simulink model "sim_flexible_unsteady_indi_turbulence"  (R2018b)
settings: Solver=ode4  StartTime=0.0  StopTime=12  FixedStep=1/600  RelTol=1e-2  AbsTol=1e-2
model workspace (MAT data in the model file):
  Var = 0
undefined symbols (not defined in the file): aircraft, alt_ground, atmosphere, envir, g, gla_indi, ic, jystck
libraries: simulink x3, atmosphere_lib x2, se2a_controller_lib x2, InputBlocks_library x2, flight_dynamics_models x1, sensors_lib x1, se2a_command_lib x1, joystick_lib x1, dspnetwork x1, flexiFlightVis_lib x1, aeroelasticity_lib x1
settings Model: EnablePacing=on  PacingRate=0.100000  ParamWorkspaceSource=ReferencedWorkspace  TunableVars=test_val  TunableVarsStorageClass=ExportedGlobal  Creator=Yannic  LastModifiedBy=yannic
settings DataIOCC: ExternalInput=[0,tp_indi.Input']  InitialState=tp_indi.State  LoadExternalInput=on  LoadInitialState=on

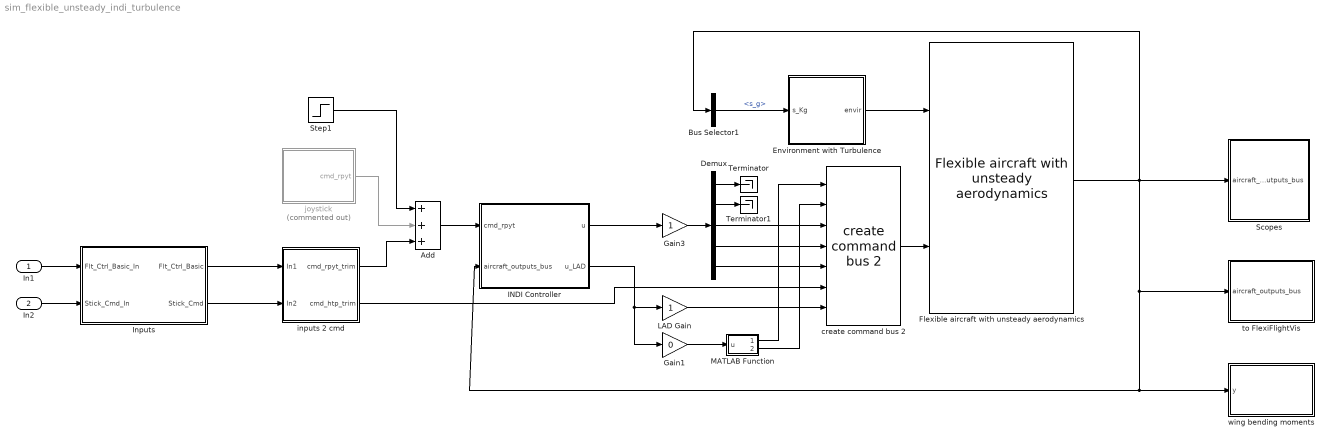
== system sim_flexible_unsteady_indi_turbulence ==
  In1 : Inport
  In2 : Inport  Port=2
  Add : Sum  Inputs=+++
  Bus Selector1 : BusSelector  OutputSignals=flexible_body_bus.rigidBodyBus.s_g
  Demux : Demux  Outputs=5
  Environment with Turbulence : Subsystem  mask{envir=envir, wind_input=2, F_g=0, gustGradDist=100, Delta_gustGradDist=100, Delta_time=3, time_0=1}
      mask prompts: envir "environment struct"; wind_input "Switch wing model (1=disable, 2=1-cos gust)"; F_g "Flight profile alleviation factor"; gustGradDist "Initial gust gradient distance, in ft"; Delta_gustGradDist "Delta gust gradient distance, in ft"; Delta_time "Time between gusts, in s"; time_0 "Time of first gust, in s"
      mask DialogControl DescGroupVar Prompt: Environment with successive 1-cos gusts
      mask DialogControl DescTextVar Prompt: Note that for the local gust delays the following structs must be in the base workspace: wing_main, wing_htp, wing_vtp, fuselage
  Flexible aircraft with unsteady aerodynamics : flight_dynamics_models/Flexible aircraft with unsteady aerodynamics  aircraft=aircraft  ic=ic
      settings: SourceProductName=SE2A library
  Gain1 : Gain  Gain=0
  Gain3 : Gain
  INDI Controller : Subsystem
  Inputs : Subsystem
  LAD Gain : Gain
  MATLAB Function : MATLAB Function  TreatAsAtomicUnit=on
  Scopes : Subsystem
  Step1 : Step  Before=zeros(4,1)  After=[0;0.05;0;0]*0  SampleTime=0
  Terminator : Terminator
  Terminator1 : Terminator
  create command bus 2 : se2a_command_lib/create command bus 2
      settings: SourceProductName=SE2A library
  inputs 2 cmd : Subsystem
  joystick : Subsystem  Commented=on
  to FlexiFlightVis : Subsystem
  wing bending moments : Subsystem
  wires:
  Environment with Turbulence/1(envir) -> Flexible aircraft with unsteady aerodynamics/1
  create command bus 2/1 -> Flexible aircraft with unsteady aerodynamics/2
  Bus Selector1/1 -> Environment with Turbulence/1(s_Kg)  "<s_g>"
  Flexible aircraft with unsteady aerodynamics/1 -> to FlexiFlightVis/1(aircraft_outputs_bus), INDI Controller/2(aircraft_outputs_bus), wing bending moments/1(y), Scopes/1(aircraft_outputs_bus), Bus Selector1/1
  joystick/1(cmd_rpyt) -> Add/2
  Demux/1 -> Terminator/1
  Demux/2 -> Terminator1/1
  Demux/3 -> create command bus 2/3
  Demux/4 -> create command bus 2/4
  Demux/5 -> create command bus 2/5
  inputs 2 cmd/2(cmd_htp_trim) -> create command bus 2/6
  In1/1 -> Inputs/1(Flt_Ctrl_Basic_In)
  In2/1 -> Inputs/2(Stick_Cmd_In)
  Inputs/1(Flt_Ctrl_Basic) -> inputs 2 cmd/1(In1)
  Inputs/2(Stick_Cmd) -> inputs 2 cmd/2(In2)
  Add/1 -> INDI Controller/1(cmd_rpyt)
  inputs 2 cmd/1(cmd_rpyt_trim) -> Add/3
  INDI Controller/1(u) -> Gain3/1
  Gain3/1 -> Demux/1
  INDI Controller/2(u_LAD) -> Gain1/1, LAD Gain/1
  MATLAB Function/1(a_l) -> create command bus 2/1
  MATLAB Function/2(a_r) -> create command bus 2/2
  Step1/1 -> Add/1
  Gain1/1 -> MATLAB Function/1(u)
  LAD Gain/1 -> create command bus 2/7

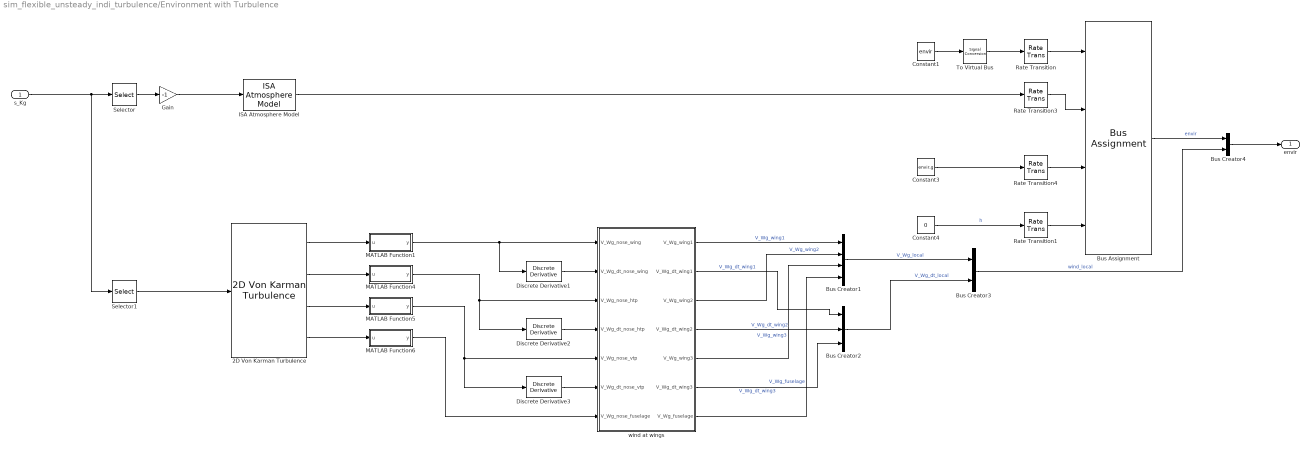
== system sim_flexible_unsteady_indi_turbulence/Environment with Turbulence ==
  s_Kg : Inport
  2D Von Karman Turbulence : atmosphere_lib/2D Von Karman Turbulence  x_max=10000  y_max=2*762  Delta_x=1  Delta_y=1  sigma=6.5  L=762  Y={aircraft.wing_main.geometry.ctrl_pt.pos(2,:),aircraft.wing_htp.geometry.ctrl_pt.pos(2,:),aircraft.wing_vtp.geometry.ctrl_pt.pos(2,:),0}  is_symmetric=on  seed=2
      settings: SourceProductName=LADAC
  Bus Assignment : BusAssignment  AssignedSignals=atmosphere,g,alt_ground
  Bus Creator1 : BusCreator  Inputs=4
  Bus Creator2 : BusCreator  Inputs=3
  Bus Creator3 : BusCreator  Inputs=2
  Bus Creator4 : BusCreator  Inputs=2
  Constant1 : Constant  Value=envir  OutDataTypeStr=Bus: envirBus
  Constant3 : Constant  Value=envir.g
  Constant4 : Constant  Value=0
  Discrete Derivative1 : simulink/Discrete/Discrete Derivative  gainval=1.0  ICPrevScaledInput=0.0  OutMin=[]  OutMax=[]  OutDataType=fixdt(1, 16)  OutScaling=2^-10  DoSatur=off
  Discrete Derivative2 : simulink/Discrete/Discrete Derivative  gainval=1.0  ICPrevScaledInput=0.0  OutMin=[]  OutMax=[]  OutDataType=fixdt(1, 16)  OutScaling=2^-10  DoSatur=off
  Discrete Derivative3 : simulink/Discrete/Discrete Derivative  gainval=1.0  ICPrevScaledInput=0.0  OutMin=[]  OutMax=[]  OutDataType=fixdt(1, 16)  OutScaling=2^-10  DoSatur=off
  Gain : Gain  Gain=-1
  ISA Atmosphere Model : atmosphere_lib/ISA Atmosphere Model
      settings: SourceProductName=LADAC
  MATLAB Function1 : MATLAB Function  TreatAsAtomicUnit=on
  MATLAB Function4 : MATLAB Function  TreatAsAtomicUnit=on
  MATLAB Function5 : MATLAB Function  TreatAsAtomicUnit=on
  MATLAB Function6 : MATLAB Function  TreatAsAtomicUnit=on
  Rate Transition{,1,3..4} (4 alike) : RateTransition
  Selector : Selector  InputPortWidth=3  IndexOptions=Index vector (dialog)  Indices=3  OutputSizes=1
  Selector1 : Selector  InputPortWidth=3  IndexOptions=Index vector (dialog)  Indices=1  OutputSizes=1
  To Virtual Bus : SignalConversion  ConversionOutput=Virtual bus  OverrideOpt=off
  wind at wings : Subsystem  mask{aircraft=aircraft, V_A=norm(ic.V_Kb,2)}
      mask prompts: aircraft "Aircraft parameters struct, see aircraftSe2aCreate"; V_A "Airspeed (TAS) in m/s"
      mask init:
      | Delta_time_main_wing = abs(aircraft.wing_main.params.x+aircraft.wing_main.geometry.ctrl_pt.pos(1,:))/V_A;
      | Delta_time_htp = abs(aircraft.wing_htp.params.x+aircraft.wing_htp.geometry.ctrl_pt.pos(1,:))/V_A;
      | Delta_time_vtp = abs(aircraft.wing_vtp.params.x+aircraft.wing_vtp.geometry.ctrl_pt.pos(1,:))/V_A;
      | Delta_time_fuse = abs(aircraft.fuselage.geometry.border_pos(1,:))/V_A;
  envir : Outport
  wires:
  wind at wings/7(V_Wg_fuselage) -> Bus Creator1/4  "V_Wg_fuselage"
  Selector/1 -> Gain/1
  s_Kg/1 -> Selector1/1, Selector/1
  To Virtual Bus/1 -> Rate Transition/1
  Bus Creator4/1 -> envir/1
  Bus Creator3/1 -> Bus Creator4/2  "wind_local"
  Bus Creator2/1 -> Bus Creator3/2  "V_Wg_dt_local"
  wind at wings/2(V_Wg_dt_wing1) -> Bus Creator2/1  "V_Wg_dt_wing1"
  wind at wings/4(V_Wg_dt_wing2) -> Bus Creator2/2  "V_Wg_dt_wing2"
  wind at wings/6(V_Wg_dt_wing3) -> Bus Creator2/3  "V_Wg_dt_wing3"
  Bus Creator1/1 -> Bus Creator3/1  "V_Wg_local"
  wind at wings/5(V_Wg_wing3) -> Bus Creator1/3  "V_Wg_wing3"
  wind at wings/3(V_Wg_wing2) -> Bus Creator1/2  "V_Wg_wing2"
  wind at wings/1(V_Wg_wing1) -> Bus Creator1/1  "V_Wg_wing1"
  Constant3/1 -> Rate Transition4/1
  Rate Transition4/1 -> Bus Assignment/3
  Gain/1 -> ISA Atmosphere Model/1
  Constant1/1 -> To Virtual Bus/1
  Rate Transition1/1 -> Bus Assignment/4
  ISA Atmosphere Model/1 -> Rate Transition3/1
  Rate Transition/1 -> Bus Assignment/1
  Bus Assignment/1 -> Bus Creator4/1  "envir"
  Rate Transition3/1 -> Bus Assignment/2
  Constant4/1 -> Rate Transition1/1  "h"
  Selector1/1 -> 2D Von Karman Turbulence/1
  2D Von Karman Turbulence/1 -> MATLAB Function1/1(u)
  MATLAB Function1/1(y) -> wind at wings/1(V_Wg_nose_wing), Discrete Derivative1/1
  Discrete Derivative1/1 -> wind at wings/2(V_Wg_dt_nose_wing)
  2D Von Karman Turbulence/2 -> MATLAB Function4/1(u)
  MATLAB Function4/1(y) -> Discrete Derivative2/1, wind at wings/3(V_Wg_nose_htp)
  2D Von Karman Turbulence/3 -> MATLAB Function5/1(u)
  MATLAB Function5/1(y) -> wind at wings/5(V_Wg_nose_vtp), Discrete Derivative3/1
  2D Von Karman Turbulence/4 -> MATLAB Function6/1(u)
  MATLAB Function6/1(y) -> wind at wings/7(V_Wg_nose_fuselage)
  Discrete Derivative2/1 -> wind at wings/4(V_Wg_dt_nose_htp)
  Discrete Derivative3/1 -> wind at wings/6(V_Wg_dt_nose_vtp)

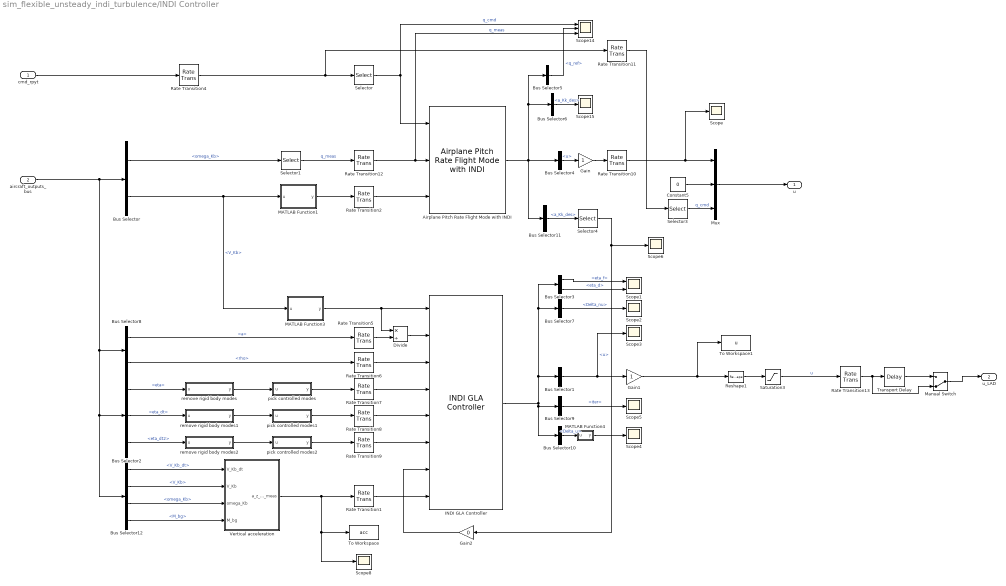
== system sim_flexible_unsteady_indi_turbulence/INDI Controller ==
  cmd_rpyt : Inport
  aircraft_outputs_bus : Inport  Port=2
  Airplane Pitch Rate Flight Mode with INDI : se2a_controller_lib/Airplane Pitch Rate Flight Mode with INDI  fm=pitch_rate_controller
  Bus Selector : BusSelector  OutputSignals=flexible_body_bus.rigidBodyBus.omega_Kb,flexible_body_bus.rigidBodyBus.V_Kb
  Bus Selector1 : BusSelector  OutputSignals=u
  Bus Selector10 : BusSelector  OutputSignals=Delta_u
  Bus Selector11 : BusSelector  OutputSignals=direct_lift_control.a_Kk_des
  Bus Selector12 : BusSelector  OutputSignals=flexible_body_bus.rigidBodyBus.V_Kb_dt,flexible_body_bus.rigidBodyBus.V_Kb,flexible_body_bus.rigidBodyBus.omega_Kb,flexible_body_bus.rigidBodyBus.M_bg
  Bus Selector2 : BusSelector  OutputSignals=flexible_body_bus.eta,flexible_body_bus.eta_dt,flexible_body_bus.eta_dt2
  Bus Selector3 : BusSelector  OutputSignals=measure.eta_f,desired.eta_d
  Bus Selector4 : BusSelector  OutputSignals=u
  Bus Selector5 : BusSelector  OutputSignals=pitch_rate_control.reference.q_ref
  Bus Selector6 : BusSelector  OutputSignals=direct_lift_control.a_Kk_des
  Bus Selector7 : BusSelector  OutputSignals=pseudo_cntrl.Delta_nu
  Bus Selector8 : BusSelector  OutputSignals=aeroBus.main.external.atmosphere.a,aeroBus.main.external.atmosphere.rho
  Bus Selector9 : BusSelector  OutputSignals=iter
  Constant5 : Constant  Value=0
  Divide : Product  Inputs=*/
  Gain : Gain
  Gain1 : Gain
  Gain2 : Gain  Gain=0
  INDI GLA Controller : se2a_controller_lib/INDI GLA Controller  gla_indi=gla_indi
  MATLAB Function1 : MATLAB Function  TreatAsAtomicUnit=on
  MATLAB Function3 : MATLAB Function  TreatAsAtomicUnit=on
  MATLAB Function4 : MATLAB Function  TreatAsAtomicUnit=on
  Manual Switch : ManualSwitch  CurrentSetting=0
  Mux : Mux  Inputs=3
  Rate Transition{1,5..9} (6 alike) : RateTransition  OutPortSampleTime=gla_indi.ts
  Rate Transition{2,4,10..13} (6 alike) : RateTransition
  Reshape1 : Reshape
  Saturation3 : Saturate  UpperLimit=gla_indi.ca.u_max  LowerLimit=gla_indi.ca.u_min
  Scope{,2..6,8,15} (8 alike) : Scope
  Scope1 : Scope  NumInputPorts=2
  Scope14 : Scope  NumInputPorts=3
  Selector : Selector  InputPortWidth=4  IndexOptions=Index vector (dialog)  Indices=2  OutputSizes=1
  Selector1 : Selector  InputPortWidth=3  IndexOptions=Index vector (dialog)  Indices=2  OutputSizes=1
  Selector3 : Selector  InputPortWidth=4  IndexOptions=Index vector (dialog)  Indices=4  OutputSizes=1
  Selector4 : Selector  InputPortWidth=3  IndexOptions=Index vector (dialog)  Indices=3  OutputSizes=1
  To Workspace : ToWorkspace  VariableName=acc  SaveFormat=Timeseries  SampleTime=-1
  To Workspace1 : ToWorkspace  VariableName=u  SaveFormat=Timeseries  SampleTime=-1
  Transport Delay : TransportDelay  DelayTime=gla_indi.ts  TransDelayFeedthrough=on
  Vertical acceleration : Subsystem
  pick controlled modes : MATLAB Function  TreatAsAtomicUnit=on
  pick controlled modes1 : MATLAB Function  TreatAsAtomicUnit=on
  pick controlled modes2 : MATLAB Function  TreatAsAtomicUnit=on
  remove rigid body modes : MATLAB Function  TreatAsAtomicUnit=on
  remove rigid body modes1 : MATLAB Function  TreatAsAtomicUnit=on
  remove rigid body modes2 : MATLAB Function  TreatAsAtomicUnit=on
  u : Outport
  u_LAD : Outport  Port=2
  wires:
  cmd_rpyt/1 -> Rate Transition4/1
  aircraft_outputs_bus/1 -> Bus Selector12/1, Bus Selector2/1, Bus Selector8/1, Bus Selector/1
  Bus Selector/1 -> Selector1/1  "<omega_Kb>"
  Bus Selector/2 -> MATLAB Function3/1(u), MATLAB Function1/1(u)  "<V_Kb>"
  Rate Transition2/1 -> Airplane Pitch Rate Flight Mode with INDI/3
  Rate Transition4/1 -> Rate Transition11/1, Selector/1
  Bus Selector4/1 -> Gain/1  "<u>"
  Rate Transition10/1 -> Scope/1, Mux/1
  Constant5/1 -> Mux/2
  Bus Selector5/1 -> Scope14/2  "<q_ref>"
  Selector/1 -> Airplane Pitch Rate Flight Mode with INDI/1, Scope14/1  "q_cmd"
  Bus Selector6/1 -> Scope15/1  "<a_Kk_des>"
  Rate Transition12/1 -> Airplane Pitch Rate Flight Mode with INDI/2, Scope14/3  "q_meas"
  Airplane Pitch Rate Flight Mode with INDI/1 -> Bus Selector5/1, Bus Selector6/1, Bus Selector11/1, Bus Selector4/1
  Mux/1 -> u/1
  Bus Selector2/1 -> remove rigid body modes/1(u)  "<eta>"
  INDI GLA Controller/1 -> Bus Selector10/1, Bus Selector9/1, Bus Selector7/1, Bus Selector3/1, Bus Selector1/1
  Bus Selector2/2 -> remove rigid body modes1/1(u)  "<eta_dt>"
  Bus Selector2/3 -> remove rigid body modes2/1(u)  "<eta_dt2>"
  Bus Selector1/1 -> Scope3/1, Gain1/1  "<u>"
  Bus Selector3/1 -> Scope1/1  "<eta_f>"
  Bus Selector3/2 -> Scope1/2  "<eta_d>"
  Gain/1 -> Rate Transition10/1
  remove rigid body modes/1(y) -> pick controlled modes/1(u)
  remove rigid body modes1/1(y) -> pick controlled modes1/1(u)
  remove rigid body modes2/1(y) -> pick controlled modes2/1(u)
  Bus Selector7/1 -> Scope2/1  "<Delta_nu>"
  Bus Selector8/2 -> Rate Transition6/1  "<rho>"
  Bus Selector8/1 -> Rate Transition5/1  "<a>"
  Bus Selector9/1 -> Scope5/1  "<iter>"
  Divide/1 -> INDI GLA Controller/2
  Rate Transition5/1 -> Divide/2
  Rate Transition6/1 -> INDI GLA Controller/3
  Rate Transition7/1 -> INDI GLA Controller/4
  Rate Transition8/1 -> INDI GLA Controller/5
  Rate Transition9/1 -> INDI GLA Controller/6
  Selector3/1 -> Mux/3  "q_cmd"
  Rate Transition11/1 -> Selector3/1
  Rate Transition13/1 -> Manual Switch/2, Transport Delay/1
  Gain1/1 -> To Workspace1/1, Reshape1/1
  Transport Delay/1 -> Manual Switch/1
  Reshape1/1 -> Saturation3/1
  Bus Selector10/1 -> MATLAB Function4/1(u)  "<Delta_u>"
  MATLAB Function4/1(y) -> Scope4/1
  Saturation3/1 -> Rate Transition13/1  "u"
  Bus Selector11/1 -> Selector4/1  "<a_Kk_des>"
  Selector4/1 -> Scope6/1, Gain2/1
  pick controlled modes/1(y) -> Rate Transition7/1
  pick controlled modes1/1(y) -> Rate Transition8/1
  pick controlled modes2/1(y) -> Rate Transition9/1
  Manual Switch/1 -> u_LAD/1
  Selector1/1 -> Rate Transition12/1  "q_meas"
  MATLAB Function3/1(y) -> INDI GLA Controller/1, Divide/1
  Gain2/1 -> INDI GLA Controller/7
  MATLAB Function1/1(y) -> Rate Transition2/1
  Bus Selector12/1 -> Vertical acceleration/1(V_Kb_dt)  "<V_Kb_dt>"
  Bus Selector12/2 -> Vertical acceleration/2(V_Kb)  "<V_Kb>"
  Bus Selector12/3 -> Vertical acceleration/3(omega_Kb)  "<omega_Kb>"
  Bus Selector12/4 -> Vertical acceleration/4(M_bg)  "<M_bg>"
  Vertical acceleration/1(a_z_Kb_meas) -> Scope8/1, To Workspace/1, Rate Transition1/1
  Rate Transition1/1 -> INDI GLA Controller/8

== system sim_flexible_unsteady_indi_turbulence/Inputs ==
  Flt_Ctrl_Basic_In : Inport
  Stick_Cmd_In : Inport  Port=2
  FltCtrlBasic : InputBlocks_library/FltCtrlBasic  SystemSampleTime=-1
  StickCmd : InputBlocks_library/StickCmd  SystemSampleTime=-1
  Flt_Ctrl_Basic : Outport
  Stick_Cmd : Outport  Port=2
  wires:
  StickCmd/1 -> Stick_Cmd/1
  FltCtrlBasic/1 -> Flt_Ctrl_Basic/1
  Flt_Ctrl_Basic_In/1 -> FltCtrlBasic/1
  Stick_Cmd_In/1 -> StickCmd/1

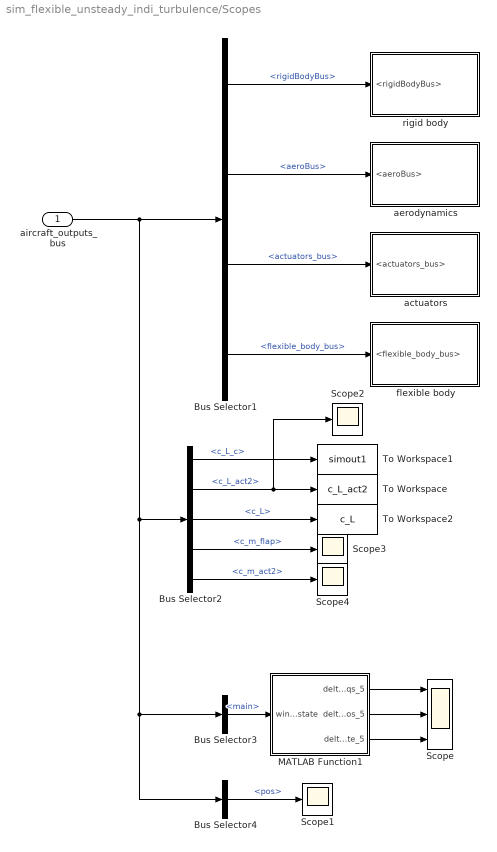
== system sim_flexible_unsteady_indi_turbulence/Scopes ==
  aircraft_outputs_bus : Inport
  Bus Selector1 : BusSelector  OutputSignals=flexible_body_bus.rigidBodyBus,aeroBus,actuators_bus,flexible_body_bus
  Bus Selector2 : BusSelector  OutputSignals=aeroBus.main.aero.unsteady.c_L_c,aeroBus.main.aero.unsteady.c_L_act2,aeroBus.main.aero.circulation.c_L,aeroBus.main.aero.unsteady.c_m_flap,aeroBus.main.aero.unsteady.c_m_act2
  Bus Selector3 : BusSelector  OutputSignals=aeroBus.main
  Bus Selector4 : BusSelector  OutputSignals=aeroBus.main.actuators.pos
  MATLAB Function1 : MATLAB Function  TreatAsAtomicUnit=on
  Scope : Scope  NumInputPorts=3
  Scope{1..4} (4 alike) : Scope
  To Workspace : ToWorkspace  VariableName=c_L_act2  SaveFormat=Timeseries  SampleTime=-1
  To Workspace1 : ToWorkspace  VariableName=simout1  SaveFormat=Timeseries  SampleTime=-1
  To Workspace2 : ToWorkspace  VariableName=c_L  SaveFormat=Timeseries  SampleTime=-1
  actuators : Subsystem
  aerodynamics : Subsystem
  flexible body : Subsystem
  rigid body : Subsystem
  wires:
  Bus Selector1/1 -> rigid body/1(<rigidBodyBus>)  "<rigidBodyBus>"
  Bus Selector1/2 -> aerodynamics/1(<aeroBus>)  "<aeroBus>"
  Bus Selector1/3 -> actuators/1(<actuators_bus>)  "<actuators_bus>"
  Bus Selector1/4 -> flexible body/1(<flexible_body_bus>)  "<flexible_body_bus>"
  MATLAB Function1/1(delta_qs_5) -> Scope/1
  MATLAB Function1/3(delta_qs_rate_5) -> Scope/3
  Bus Selector2/3 -> To Workspace2/1  "<c_L>"
  MATLAB Function1/2(delta_qs_pos_5) -> Scope/2
  Bus Selector3/1 -> MATLAB Function1/1(wing_state)  "<main>"
  Bus Selector2/2 -> Scope2/1, To Workspace/1  "<c_L_act2>"
  aircraft_outputs_bus/1 -> Bus Selector4/1, Bus Selector3/1, Bus Selector2/1, Bus Selector1/1
  Bus Selector2/1 -> To Workspace1/1  "<c_L_c>"
  Bus Selector4/1 -> Scope1/1  "<pos>"
  Bus Selector2/4 -> Scope3/1  "<c_m_flap>"
  Bus Selector2/5 -> Scope4/1  "<c_m_act2>"

== system sim_flexible_unsteady_indi_turbulence/inputs 2 cmd ==
  In1 : Inport
  In2 : Inport  Port=2
  Demux : Demux  Outputs=2
  Mux : Mux  Inputs=2
  Selector : Selector  InputPortWidth=4  IndexOptions=Index vector (dialog)  Indices=1:3  OutputSizes=1
  cmd_rpyt_trim : Outport
  cmd_htp_trim : Outport  Port=2
  wires:
  Demux/1 -> Mux/2
  Selector/1 -> Mux/1
  Mux/1 -> cmd_rpyt_trim/1
  In1/1 -> Demux/1
  Demux/2 -> cmd_htp_trim/1
  In2/1 -> Selector/1

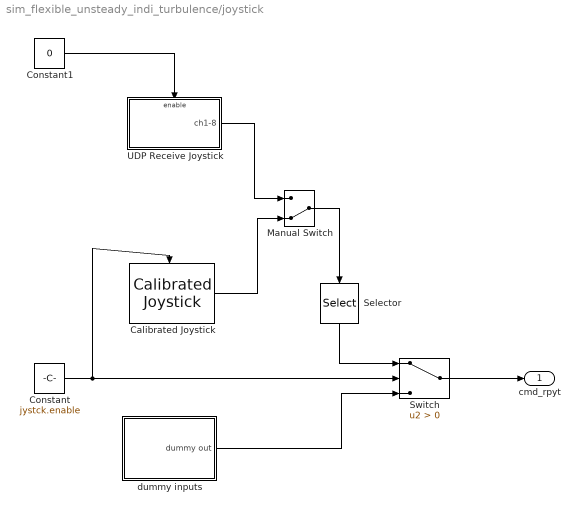
== system sim_flexible_unsteady_indi_turbulence/joystick ==
  Calibrated Joystick : joystick_lib/Calibrated Joystick  jystck=jystck
      settings: SourceProductName=LADAC
  Constant : Constant  Value=jystck.enable
  Constant1 : Constant  Value=0
  Manual Switch : ManualSwitch  CurrentSetting=0
  Selector : Selector  InputPortWidth=8  IndexOptions=Index vector (dialog)  Indices=[1,2,3,4]  OutputSizes=1
  Switch : Switch  Criteria=u2 > Threshold
  UDP Receive Joystick : Subsystem
  dummy inputs : Subsystem
  cmd_rpyt : Outport
  wires:
  Switch/1 -> cmd_rpyt/1
  Constant/1 -> Calibrated Joystick/Enable, Switch/2
  dummy inputs/1(dummy out) -> Switch/3
  Selector/1 -> Switch/1
  UDP Receive Joystick/1(ch1-8) -> Manual Switch/1
  Manual Switch/1 -> Selector/1
  Calibrated Joystick/1 -> Manual Switch/2
  Constant1/1 -> UDP Receive Joystick/Enable

== system sim_flexible_unsteady_indi_turbulence/to FlexiFlightVis ==
  aircraft_outputs_bus : Inport
  Bus Creator : BusCreator  Inputs=1
  Bus Selector : BusSelector  OutputSignals=flexible_body_bus.rigidBodyBus,aeroBus.main,aeroBus.htp,aeroBus.vtp,aeroBus.fuselage
  Constant : Constant  Value=aircraft.config.xyz_ref_c
  Send to FlexiFlightVis : flexiFlightVis_lib/Send to FlexiFlightVis  sample_time=1/120  ip_address='localhost'  ip_port=4321  wing_cell={aircraft.wing_main.state,aircraft.wing_htp.state,aircraft.wing_vtp.state}  fuse_cell={aircraft.fuselage.state}
      settings: SourceProductName=LADAC
  wires:
  aircraft_outputs_bus/1 -> Bus Selector/1
  Bus Selector/4 -> Send to FlexiFlightVis/5  "<vtp>"
  Bus Selector/5 -> Send to FlexiFlightVis/6  "<fuselage>"
  Bus Selector/3 -> Send to FlexiFlightVis/4  "<htp>"
  Bus Selector/2 -> Send to FlexiFlightVis/3  "<main>"
  Bus Selector/1 -> Send to FlexiFlightVis/1  "<rigidBodyBus>"
  Constant/1 -> Bus Creator/1  "xyz_ref_c"
  Bus Creator/1 -> Send to FlexiFlightVis/2

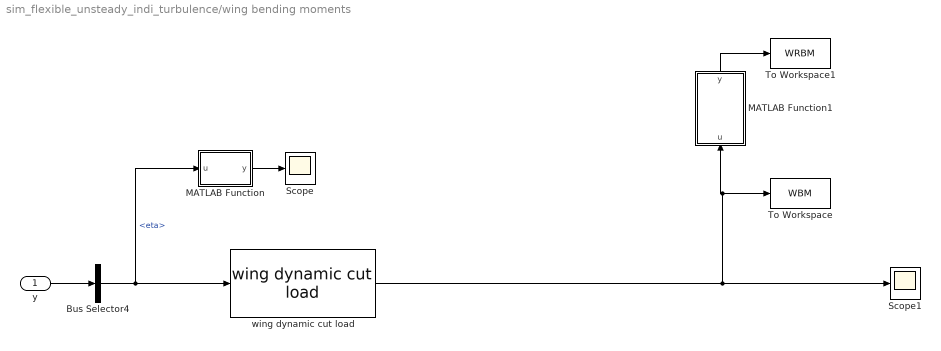
== system sim_flexible_unsteady_indi_turbulence/wing bending moments ==
  y : Inport
  Bus Selector4 : BusSelector  OutputSignals=flexible_body_bus.eta
  MATLAB Function : MATLAB Function  TreatAsAtomicUnit=on
  MATLAB Function1 : MATLAB Function  TreatAsAtomicUnit=on
  Scope : Scope
  Scope1 : Scope
  To Workspace : ToWorkspace  VariableName=WBM  SaveFormat=Timeseries  SampleTime=-1
  To Workspace1 : ToWorkspace  VariableName=WRBM  SaveFormat=Timeseries  SampleTime=-1
  wing dynamic cut load : aeroelasticity_lib/wing dynamic cut load  structure=structure  structure_red=aircraft.eom_flexible.structure_red  eta=[-0.9:0.2:0.9]  popup_index_1=Mx  popup_index_2=reverse_right
      settings: SourceProductName=LADAC
  wires:
  Bus Selector4/1 -> wing dynamic cut load/1, MATLAB Function/1(u)  "<eta>"
  y/1 -> Bus Selector4/1
  wing dynamic cut load/1 -> To Workspace/1, MATLAB Function1/1(u), Scope1/1
  MATLAB Function/1(y) -> Scope/1
  MATLAB Function1/1(y) -> To Workspace1/1

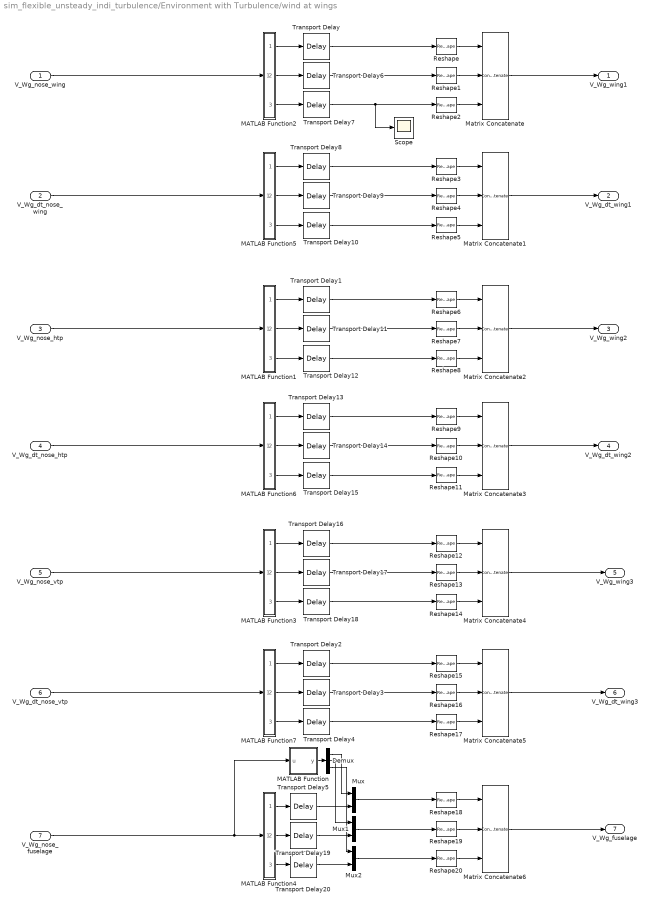
== system sim_flexible_unsteady_indi_turbulence/Environment with Turbulence/wind at wings ==
  V_Wg_nose_wing : Inport
  V_Wg_dt_nose_wing : Inport  Port=2
  V_Wg_nose_htp : Inport  Port=3
  V_Wg_dt_nose_htp : Inport  Port=4
  V_Wg_nose_vtp : Inport  Port=5
  V_Wg_dt_nose_vtp : Inport  Port=6
  V_Wg_nose_fuselage : Inport  Port=7
  Demux : Demux  Outputs=3
  MATLAB Function : MATLAB Function  TreatAsAtomicUnit=on
  MATLAB Function1 : MATLAB Function  TreatAsAtomicUnit=on
  MATLAB Function2 : MATLAB Function  TreatAsAtomicUnit=on
  MATLAB Function3 : MATLAB Function  TreatAsAtomicUnit=on
  MATLAB Function4 : MATLAB Function  TreatAsAtomicUnit=on
  MATLAB Function5 : MATLAB Function  TreatAsAtomicUnit=on
  MATLAB Function6 : MATLAB Function  TreatAsAtomicUnit=on
  MATLAB Function7 : MATLAB Function  TreatAsAtomicUnit=on
  Matrix Concatenate{,1..6} (7 alike) : Concatenate  NumInputs=3  Mode=Multidimensional array
  Mux : Mux  Inputs=2
  Mux1 : Mux  Inputs=2
  Mux2 : Mux  Inputs=2
  Reshape{,1..20} (21 alike) : Reshape  OutputDimensionality=Row vector (2-D)
  Scope : Scope
  Transport Delay{,6..10} (6 alike) : TransportDelay  DelayTime=Delta_time_main_wing
  Transport Delay{1,11..15} (6 alike) : TransportDelay  DelayTime=Delta_time_htp
  Transport Delay{2..4,16..18} (6 alike) : TransportDelay  DelayTime=Delta_time_vtp
  Transport Delay19 : TransportDelay  DelayTime=Delta_time_fuse(2:end)
  Transport Delay20 : TransportDelay  DelayTime=Delta_time_fuse(2:end)
  Transport Delay5 : TransportDelay  DelayTime=Delta_time_fuse(2:end)
  V_Wg_wing1 : Outport
  V_Wg_dt_wing1 : Outport  Port=2
  V_Wg_wing2 : Outport  Port=3
  V_Wg_dt_wing2 : Outport  Port=4
  V_Wg_wing3 : Outport  Port=5
  V_Wg_dt_wing3 : Outport  Port=6
  V_Wg_fuselage : Outport  Port=7
  wires:
  Reshape20/1 -> Matrix Concatenate6/3
  Reshape19/1 -> Matrix Concatenate6/2
  Reshape18/1 -> Matrix Concatenate6/1
  Reshape17/1 -> Matrix Concatenate5/3
  Reshape16/1 -> Matrix Concatenate5/2
  Reshape15/1 -> Matrix Concatenate5/1
  Reshape14/1 -> Matrix Concatenate4/3
  Reshape13/1 -> Matrix Concatenate4/2
  Reshape12/1 -> Matrix Concatenate4/1
  Reshape11/1 -> Matrix Concatenate3/3
  Reshape10/1 -> Matrix Concatenate3/2
  Reshape9/1 -> Matrix Concatenate3/1
  Reshape8/1 -> Matrix Concatenate2/3
  Reshape7/1 -> Matrix Concatenate2/2
  Reshape6/1 -> Matrix Concatenate2/1
  Reshape5/1 -> Matrix Concatenate1/3
  Reshape4/1 -> Matrix Concatenate1/2
  Reshape3/1 -> Matrix Concatenate1/1
  Reshape2/1 -> Matrix Concatenate/3
  Reshape1/1 -> Matrix Concatenate/2
  Reshape/1 -> Matrix Concatenate/1
  V_Wg_nose_htp/1 -> MATLAB Function1/1(V)
  V_Wg_dt_nose_wing/1 -> MATLAB Function5/1(V)
  MATLAB Function2/1(u) -> Transport Delay/1
  MATLAB Function2/2(v) -> Transport Delay6/1
  MATLAB Function2/3(w) -> Transport Delay7/1
  Transport Delay6/1 -> Reshape1/1
  Transport Delay7/1 -> Scope/1, Reshape2/1
  Matrix Concatenate/1 -> V_Wg_wing1/1
  Transport Delay/1 -> Reshape/1
  MATLAB Function5/2(v) -> Transport Delay9/1
  Transport Delay10/1 -> Reshape5/1
  Transport Delay9/1 -> Reshape4/1
  MATLAB Function5/3(w) -> Transport Delay10/1
  MATLAB Function5/1(u) -> Transport Delay8/1
  Matrix Concatenate1/1 -> V_Wg_dt_wing1/1
  Transport Delay8/1 -> Reshape3/1
  MATLAB Function1/1(u) -> Transport Delay1/1
  MATLAB Function1/2(v) -> Transport Delay11/1
  MATLAB Function1/3(w) -> Transport Delay12/1
  Transport Delay12/1 -> Reshape8/1
  Transport Delay11/1 -> Reshape7/1
  Transport Delay1/1 -> Reshape6/1
  Matrix Concatenate2/1 -> V_Wg_wing2/1
  Transport Delay13/1 -> Reshape9/1
  Transport Delay14/1 -> Reshape10/1
  Transport Delay15/1 -> Reshape11/1
  MATLAB Function6/3(w) -> Transport Delay15/1
  MATLAB Function6/2(v) -> Transport Delay14/1
  MATLAB Function6/1(u) -> Transport Delay13/1
  Matrix Concatenate3/1 -> V_Wg_dt_wing2/1
  MATLAB Function3/1(u) -> Transport Delay16/1
  MATLAB Function3/2(v) -> Transport Delay17/1
  MATLAB Function3/3(w) -> Transport Delay18/1
  Transport Delay18/1 -> Reshape14/1
  Transport Delay17/1 -> Reshape13/1
  Transport Delay16/1 -> Reshape12/1
  Matrix Concatenate4/1 -> V_Wg_wing3/1
  MATLAB Function7/2(v) -> Transport Delay3/1
  Transport Delay3/1 -> Reshape16/1
  Transport Delay2/1 -> Reshape15/1
  MATLAB Function7/1(u) -> Transport Delay2/1
  MATLAB Function7/3(w) -> Transport Delay4/1
  Transport Delay4/1 -> Reshape17/1
  Matrix Concatenate5/1 -> V_Wg_dt_wing3/1
  Matrix Concatenate6/1 -> V_Wg_fuselage/1
  Transport Delay20/1 -> Mux2/2
  MATLAB Function4/3(w) -> Transport Delay20/1
  MATLAB Function4/1(u) -> Transport Delay5/1
  Transport Delay5/1 -> Mux/2
  Transport Delay19/1 -> Mux1/2
  MATLAB Function4/2(v) -> Transport Delay19/1
  Mux/1 -> Reshape18/1
  Mux1/1 -> Reshape19/1
  Mux2/1 -> Reshape20/1
  MATLAB Function/1(y) -> Demux/1
  Demux/1 -> Mux/1
  Demux/2 -> Mux1/1
  Demux/3 -> Mux2/1
  V_Wg_nose_wing/1 -> MATLAB Function2/1(V)
  V_Wg_dt_nose_htp/1 -> MATLAB Function6/1(V)
  V_Wg_nose_vtp/1 -> MATLAB Function3/1(V)
  V_Wg_dt_nose_vtp/1 -> MATLAB Function7/1(V)
  V_Wg_nose_fuselage/1 -> MATLAB Function/1(u), MATLAB Function4/1(V)

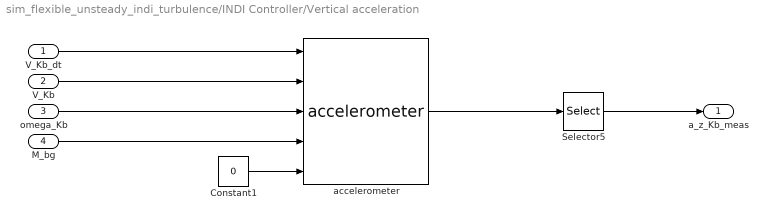
== system sim_flexible_unsteady_indi_turbulence/INDI Controller/Vertical acceleration ==
  V_Kb_dt : Inport
  V_Kb : Inport  Port=2
  omega_Kb : Inport  Port=3
  M_bg : Inport  Port=4
  Constant1 : Constant  Value=0  VectorParams1D=off
  Selector5 : Selector  InputPortWidth=3  IndexOptions=Index vector (dialog)  Indices=3  OutputSizes=1
  accelerometer : sensors_lib/accelerometer  SystemSampleTime=-1
      settings: SourceProductName=LADAC
  a_z_Kb_meas : Outport
  wires:
  M_bg/1 -> accelerometer/4
  Selector5/1 -> a_z_Kb_meas/1
  accelerometer/1 -> Selector5/1
  V_Kb/1 -> accelerometer/2
  omega_Kb/1 -> accelerometer/3
  V_Kb_dt/1 -> accelerometer/1
  Constant1/1 -> accelerometer/5

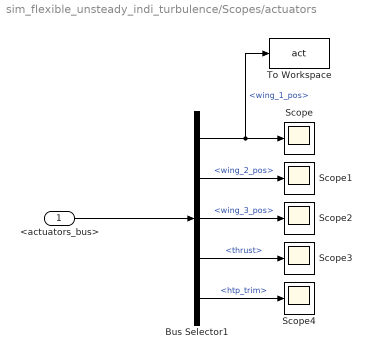
== system sim_flexible_unsteady_indi_turbulence/Scopes/actuators ==
  <actuators_bus> : Inport
  Bus Selector1 : BusSelector  OutputSignals=wing_1_pos,wing_2_pos,wing_3_pos,thrust,htp_trim
  Scope{,1..4} (5 alike) : Scope
  To Workspace : ToWorkspace  VariableName=act  SaveFormat=Timeseries  SampleTime=-1
  wires:
  <actuators_bus>/1 -> Bus Selector1/1
  Bus Selector1/1 -> To Workspace/1, Scope/1  "<wing_1_pos>"
  Bus Selector1/2 -> Scope1/1  "<wing_2_pos>"
  Bus Selector1/3 -> Scope2/1  "<wing_3_pos>"
  Bus Selector1/4 -> Scope3/1  "<thrust>"
  Bus Selector1/5 -> Scope4/1  "<htp_trim>"

== system sim_flexible_unsteady_indi_turbulence/Scopes/aerodynamics ==
  <aeroBus> : Inport
  Bus Selector1 : BusSelector  OutputSignals=main,htp,vtp
  htp : Subsystem
  vtp : Subsystem
  wing : Subsystem
  wires:
  <aeroBus>/1 -> Bus Selector1/1
  Bus Selector1/2 -> htp/1(htp)  "<htp>"
  Bus Selector1/1 -> wing/1(main)  "<main>"
  Bus Selector1/3 -> vtp/1(vtp)  "<vtp>"

== system sim_flexible_unsteady_indi_turbulence/Scopes/flexible body ==
  <flexible_body_bus> : Inport
  Bus Selector1 : BusSelector  OutputSignals=eta,eta_dt,eta_dt2,generalized_load_vector
  Scope{,1..3} (4 alike) : Scope
  To Workspace : ToWorkspace  VariableName=eta  SaveFormat=Timeseries  SampleTime=-1
  wires:
  Bus Selector1/4 -> Scope3/1  "<generalized_load_vector>"
  Bus Selector1/3 -> Scope2/1  "<eta_dt2>"
  Bus Selector1/2 -> Scope1/1  "<eta_dt>"
  Bus Selector1/1 -> To Workspace/1, Scope/1  "<eta>"
  <flexible_body_bus>/1 -> Bus Selector1/1

== system sim_flexible_unsteady_indi_turbulence/Scopes/rigid body ==
  <rigidBodyBus> : Inport
  Bus Selector : BusSelector  OutputSignals=V_Kb_dt,V_Kg,omega_Kb_dt,omega_Kb,EulerAngles,s_g
  Scope{,1..5} (6 alike) : Scope
  wires:
  Bus Selector/5 -> Scope/1  "<EulerAngles>"
  Bus Selector/2 -> Scope1/1  "<V_Kg>"
  Bus Selector/6 -> Scope3/1  "<s_g>"
  Bus Selector/4 -> Scope2/1  "<omega_Kb>"
  <rigidBodyBus>/1 -> Bus Selector/1
  Bus Selector/3 -> Scope4/1  "<omega_Kb_dt>"
  Bus Selector/1 -> Scope5/1  "<V_Kb_dt>"

== system sim_flexible_unsteady_indi_turbulence/joystick/UDP Receive Joystick ==
  Enable : EnablePort
  Terminator : Terminator
  UDP Receive1 : dspnetwork/UDP Receive  localURL='0.0.0.0'  localPort=25000  remoteURL='192.168.178.2'  remotePort=-1  recvBufferSize=8*8  dims=8  signalDatatype=double  isVarSize=off  showBlockingTime=on  blockingTime=1  sampletime=1/30  blockPlatform=HOST
      settings: SourceProductName=DSP System Toolbox  SourceProductBaseCode=DS
  ch1-8 : Outport
  wires:
  UDP Receive1/1 -> ch1-8/1
  UDP Receive1/2 -> Terminator/1

== system sim_flexible_unsteady_indi_turbulence/joystick/dummy inputs ==
  Constant : Constant  Value=0
  Mux1 : Mux
  Product : Product
  Sine Wave : Sin  Amplitude=0.1  Frequency=3  SampleTime=0
  Sine Wave1 : Sin  Amplitude=0.1  Frequency=4  SampleTime=0
  Sine Wave2 : Sin  Amplitude=0.1  Frequency=5  SampleTime=0
  Step3 : Step  Time=10  Before=1  After=0  SampleTime=0
  dummy out : Outport
  wires:
  Constant/1 -> Mux1/4  "cmd_thr"
  Sine Wave2/1 -> Mux1/3  "cmd_yaw"
  Sine Wave1/1 -> Mux1/2  "cmd_pitch"
  Sine Wave/1 -> Mux1/1  "cmd_roll"
  Mux1/1 -> Product/1
  Product/1 -> dummy out/1
  Step3/1 -> Product/2  "disabler"

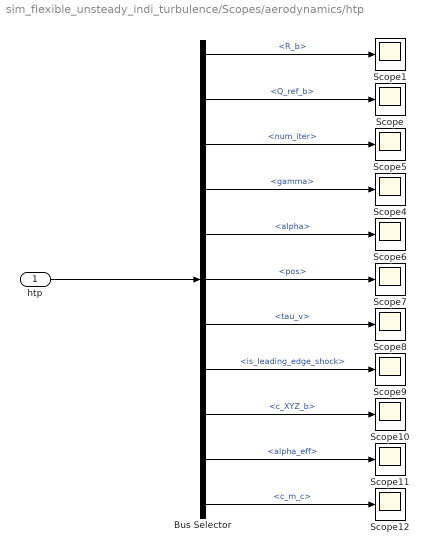
== system sim_flexible_unsteady_indi_turbulence/Scopes/aerodynamics/htp ==
  htp : Inport
  Bus Selector : BusSelector  OutputSignals=aero.force_glob.R_b,aero.force_glob.Q_ref_b,aero.circulation.num_iter,aero.circulation.gamma,body.alpha,actuators.pos,aero.unsteady.tau_v,aero.unsteady.is_leading_edge_shock,aero.coeff_loc.c_XYZ_b,aero.circulation.alpha_eff,aero.unsteady.c_m_c
  Scope{,1,4..12} (11 alike) : Scope
  wires:
  Bus Selector/11 -> Scope12/1  "<c_m_c>"
  Bus Selector/10 -> Scope11/1  "<alpha_eff>"
  Bus Selector/9 -> Scope10/1  "<c_XYZ_b>"
  Bus Selector/8 -> Scope9/1  "<is_leading_edge_shock>"
  Bus Selector/7 -> Scope8/1  "<tau_v>"
  Bus Selector/6 -> Scope7/1  "<pos>"
  Bus Selector/5 -> Scope6/1  "<alpha>"
  htp/1 -> Bus Selector/1
  Bus Selector/1 -> Scope1/1  "<R_b>"
  Bus Selector/2 -> Scope/1  "<Q_ref_b>"
  Bus Selector/4 -> Scope4/1  "<gamma>"
  Bus Selector/3 -> Scope5/1  "<num_iter>"

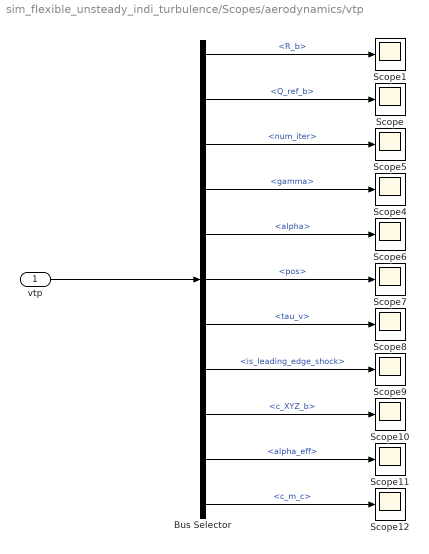
== system sim_flexible_unsteady_indi_turbulence/Scopes/aerodynamics/vtp ==
  vtp : Inport
  Bus Selector : BusSelector  OutputSignals=aero.force_glob.R_b,aero.force_glob.Q_ref_b,aero.circulation.num_iter,aero.circulation.gamma,body.alpha,actuators.pos,aero.unsteady.tau_v,aero.unsteady.is_leading_edge_shock,aero.coeff_loc.c_XYZ_b,aero.circulation.alpha_eff,aero.unsteady.c_m_c
  Scope{,1,4..12} (11 alike) : Scope
  wires:
  Bus Selector/3 -> Scope5/1  "<num_iter>"
  Bus Selector/4 -> Scope4/1  "<gamma>"
  Bus Selector/2 -> Scope/1  "<Q_ref_b>"
  Bus Selector/1 -> Scope1/1  "<R_b>"
  vtp/1 -> Bus Selector/1
  Bus Selector/5 -> Scope6/1  "<alpha>"
  Bus Selector/6 -> Scope7/1  "<pos>"
  Bus Selector/7 -> Scope8/1  "<tau_v>"
  Bus Selector/8 -> Scope9/1  "<is_leading_edge_shock>"
  Bus Selector/9 -> Scope10/1  "<c_XYZ_b>"
  Bus Selector/10 -> Scope11/1  "<alpha_eff>"
  Bus Selector/11 -> Scope12/1  "<c_m_c>"

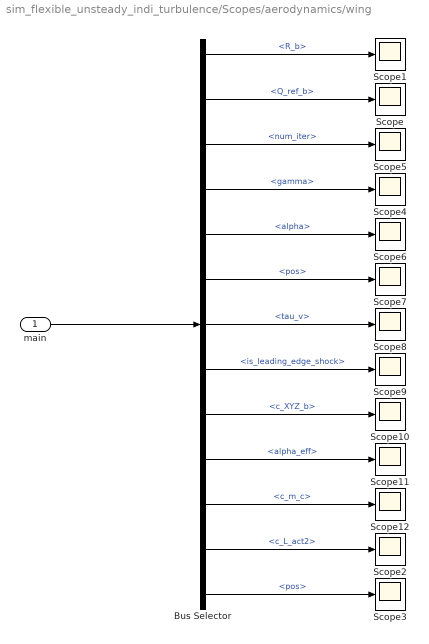
== system sim_flexible_unsteady_indi_turbulence/Scopes/aerodynamics/wing ==
  main : Inport
  Bus Selector : BusSelector  OutputSignals=aero.force_glob.R_b,aero.force_glob.Q_ref_b,aero.circulation.num_iter,aero.circulation.gamma,body.alpha,actuators.pos,aero.unsteady.tau_v,aero.unsteady.is_leading_edge_shock,aero.coeff_loc.c_XYZ_b,aero.circulation.alpha_eff,aero.unsteady.c_m_c,aero.unsteady.c_L_act2,actuators.pos
  Scope{,1..12} (13 alike) : Scope
  wires:
  Bus Selector/3 -> Scope5/1  "<num_iter>"
  Bus Selector/4 -> Scope4/1  "<gamma>"
  Bus Selector/2 -> Scope/1  "<Q_ref_b>"
  Bus Selector/1 -> Scope1/1  "<R_b>"
  main/1 -> Bus Selector/1
  Bus Selector/5 -> Scope6/1  "<alpha>"
  Bus Selector/6 -> Scope7/1  "<pos>"
  Bus Selector/7 -> Scope8/1  "<tau_v>"
  Bus Selector/8 -> Scope9/1  "<is_leading_edge_shock>"
  Bus Selector/9 -> Scope10/1  "<c_XYZ_b>"
  Bus Selector/10 -> Scope11/1  "<alpha_eff>"
  Bus Selector/11 -> Scope12/1  "<c_m_c>"
  Bus Selector/13 -> Scope3/1  "<pos>"
  Bus Selector/12 -> Scope2/1  "<c_L_act2>"

== matlab function sim_flexible_unsteady_indi_turbulence/INDI Controller/MATLAB Function3 ==
  data: u input; y output
function y = fcn(u)
y=norm(u,2);
end

== matlab function sim_flexible_unsteady_indi_turbulence/INDI Controller/pick controlled modes1 ==
  data: u input; y output; gla_indi parameter
function y = fcn(u,gla_indi)
y = u(gla_indi.mcidx);
end

== matlab function sim_flexible_unsteady_indi_turbulence/Scopes/MATLAB Function1 ==
  data: wing_state input; delta_qs_5 output; delta_qs_pos_5 output; delta_qs_rate_5 output
function [delta_qs_5,delta_qs_pos_5,delta_qs_rate_5] = fcn(wing_state)

abs_V_i = vecnorm(wing_state.aero.local_inflow.V_25,2,1);
F = airfoilFlapEffectiveness(wing_state.geometry.segments.flap_depth);
delta_qs = airfoilFlapDeltaQs( F.F_10, F.F_11,...
    abs_V_i, sum(wing_state.geometry.ctrl_pt.c,3), deg2rad(wing_state.actuators.segments.pos(2,:)), ...
    deg2rad(wing_state.actuators.segments.rate(2,:)) ) .* cos(wing_state.geometry.segments.flap_sweep);
delta_qs_pos = airfoilFlapDeltaQs( F.F_10, F.F_11,...
    abs_V_i, sum(wing_state.geometry.ctrl_pt.c,3), deg2rad(wing_state.actuators.segments.pos(2,:)), ...
    0 ) .* cos(wing_state.geometry.segments.flap_sweep);
delta_qs_rate = airfoilFlapDeltaQs( F.F_10, F.F_11,...
    abs_V_i, sum(wing_state.geometry.ctrl_pt.c,3), 0, ...
    deg2rad(wing_state.actuators.segments.rate(2,:)) ) .* cos(wing_state.geometry.segments.flap_sweep);

delta_qs_5 = delta_qs(15:19);
delta_qs_pos_5 = delta_qs_pos(15:19);
delta_qs_rate_5 = delta_qs_rate(15:19);


end

== matlab function sim_flexible_unsteady_indi_turbulence/INDI Controller/pick controlled modes2 ==
  data: u input; y output; gla_indi parameter
function y = fcn(u,gla_indi)
y = u(gla_indi.mcidx);
end

== matlab function sim_flexible_unsteady_indi_turbulence/INDI Controller/remove rigid body modes ==
  data: u input; y output
function y = fcn(u)
y = u(7:end);
end

== matlab function sim_flexible_unsteady_indi_turbulence/INDI Controller/MATLAB Function1 ==
  data: u input; y output
function y = fcn(u)
y = norm(u,2);
end

== matlab function sim_flexible_unsteady_indi_turbulence/INDI Controller/remove rigid body modes1 ==
  data: u input; y output
function y = fcn(u)
y = u(7:end);
end

== matlab function sim_flexible_unsteady_indi_turbulence/wing bending moments/MATLAB Function ==
  data: u input; y output
function y = fcn(u)

y = u(7:end);

== matlab function sim_flexible_unsteady_indi_turbulence/INDI Controller/remove rigid body modes2 ==
  data: u input; y output
function y = fcn(u)
y = u(7:end);
end

== matlab function sim_flexible_unsteady_indi_turbulence/INDI Controller/pick controlled modes ==
  data: u input; y output; gla_indi parameter
function y = fcn(u,gla_indi)
y = u(gla_indi.mcidx);
end

== matlab function sim_flexible_unsteady_indi_turbulence/Environment with Turbulence/MATLAB Function1 ==
  data: u input; y output
function y = fcn(u)

y = [zeros(2,length(u));u(:)'];
y(isnan(y))=0;

== matlab function sim_flexible_unsteady_indi_turbulence/MATLAB Function ==
  data: u input; a_l output; a_r output
function [a_l,a_r] = fcn(u)
n_u = length(u);
a_l = u(1:n_u/2);
a_r = u(n_u/2+1:end);
end

== matlab function sim_flexible_unsteady_indi_turbulence/Environment with Turbulence/wind at wings/MATLAB Function2 ==
  data: V input; u output; v output; w output
function [u,v,w] = fcn(V)

u = V(1,:);
v = V(2,:);
w = V(3,:);

== matlab function sim_flexible_unsteady_indi_turbulence/INDI Controller/MATLAB Function4 ==
  data: u input; y output
function y = fcn(u)

y = u(10);

== matlab function sim_flexible_unsteady_indi_turbulence/wing bending moments/MATLAB Function1 ==
  data: u input; y output
function y = fcn(u)
len_u = length(u);
idx = len_u/2;
y = u([idx,idx+1]);
end

== matlab function sim_flexible_unsteady_indi_turbulence/Environment with Turbulence/wind at wings/MATLAB Function1 ==
  data: V input; u output; v output; w output
function [u,v,w] = fcn(V)

u = V(1,:);
v = V(2,:);
w = V(3,:);

== matlab function sim_flexible_unsteady_indi_turbulence/Environment with Turbulence/wind at wings/MATLAB Function3 ==
  data: V input; u output; v output; w output
function [u,v,w] = fcn(V)

u = V(1,:);
v = V(2,:);
w = V(3,:);

== matlab function sim_flexible_unsteady_indi_turbulence/Environment with Turbulence/wind at wings/MATLAB Function4 ==
  data: V input; u output; v output; w output
function [u,v,w] = fcn(V)

u = V(1,:);
v = V(2,:);
w = V(3,:);

== matlab function sim_flexible_unsteady_indi_turbulence/Environment with Turbulence/wind at wings/MATLAB Function ==
  data: u input; y output
function y = fcn(u)

y = u(:,1);

== matlab function sim_flexible_unsteady_indi_turbulence/Environment with Turbulence/wind at wings/MATLAB Function5 ==
  data: V input; u output; v output; w output
function [u,v,w] = fcn(V)

u = V(1,:);
v = V(2,:);
w = V(3,:);

== matlab function sim_flexible_unsteady_indi_turbulence/Environment with Turbulence/wind at wings/MATLAB Function6 ==
  data: V input; u output; v output; w output
function [u,v,w] = fcn(V)

u = V(1,:);
v = V(2,:);
w = V(3,:);

== matlab function sim_flexible_unsteady_indi_turbulence/Environment with Turbulence/wind at wings/MATLAB Function7 ==
  data: V input; u output; v output; w output
function [u,v,w] = fcn(V)

u = V(1,:);
v = V(2,:);
w = V(3,:);

== matlab function sim_flexible_unsteady_indi_turbulence/Environment with Turbulence/MATLAB Function4 ==
  data: u input; y output
function y = fcn(u)

y = [zeros(2,length(u));u(:)'];
y(isnan(y))=0;

== matlab function sim_flexible_unsteady_indi_turbulence/Environment with Turbulence/MATLAB Function5 ==
  data: u input; y output
function y = fcn(u)

y = [zeros(2,length(u));u(:)'];
y(isnan(y))=0;

== matlab function sim_flexible_unsteady_indi_turbulence/Environment with Turbulence/MATLAB Function6 ==
  data: u input; y output
function y = fcn(u)

y = [zeros(2,length(u));u(:)'];
y(isnan(y))=0;
